simulink model "hw6_"  (Simulink 7.9)
settings: Solver=ode45  StartTime=0.0  StopTime=200.0  RelTol=1e-3
settings Model: Creator=bazkoale  LastModifiedBy=alex
settings DataIOCC: SignalLoggingSaveFormat=Dataset
settings OptimizationCC: ExpressionDepthLimit=128
settings DebuggingCC: MultiTaskDSMMsg=warning  MultiTaskCondExecSysMsg=none  StrictBusMsg=None
settings RTWCC: IncludeERTFirstTime=on
settings CodeAppCC: CustomSymbolStrType=$N$R$M_T

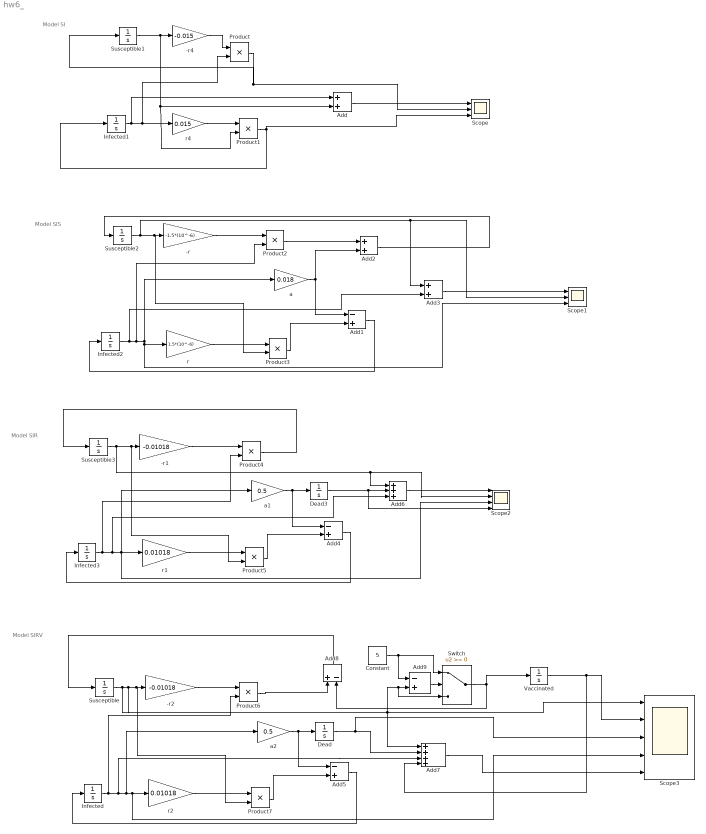
== system hw6_ ==
  note: Model SI
  note: Model SIS
  note: Model SIR
  note: Model SIRV
  -r : Gain  Gain=-1.5*(10^-6)
  -r1 : Gain  Gain=-0.01018
  -r2 : Gain  Gain=-0.01018
  -r4 : Gain  Gain=-0.015
  Add : Sum
  Add{1,4..5,9} (4 alike) : Sum  Inputs=-+
  Add2 : Sum
  Add3 : Sum
  Add6 : Sum  Inputs=+++
  Add7 : Sum  Inputs=++++
  Add8 : Sum  Inputs=+-
  Constant : Constant  Value=5
  Dead : Integrator
  Dead3 : Integrator
  Infected : Integrator  InitialCondition=1
  Infected1 : Integrator  InitialCondition=1
  Infected2 : Integrator  InitialCondition=10
  Infected3 : Integrator  InitialCondition=1
  Product{,1..7} (8 alike) : Product
  Scope : Scope  NumInputPorts=3
      settings: YMin=-5~-5~-5  YMax=5~5~5
  Scope1 : Scope  NumInputPorts=3
      settings: YMin=-5~-5~-5  YMax=5~5~5
  Scope2 : Scope  NumInputPorts=4
      settings: YMin=-5~-5~-5~-5  YMax=5~5~5~5  SaveName=ScopeData2
  Scope3 : Scope  NumInputPorts=5
      settings: YMin=-5~-5~-5~-5~-5  YMax=5~5~5~5~5  SaveName=ScopeData3
  Susceptible : Integrator  InitialCondition=99
  Susceptible1 : Integrator  InitialCondition=99
  Susceptible2 : Integrator  InitialCondition=200000-10
  Susceptible3 : Integrator  InitialCondition=99
  Switch : Switch
  Vaccinated : Integrator
  a : Gain  Gain=0.018
  a1 : Gain  Gain=0.5
  a2 : Gain  Gain=0.5
  r : Gain  Gain=1.5*(10^-6)
  r1 : Gain  Gain=0.01018
  r2 : Gain  Gain=0.01018
  r4 : Gain  Gain=0.015
  wires:
  Susceptible1/1 -> Add/2, Product1/2, -r4/1
  Infected1/1 -> Add/1, Product/2, r4/1
  Product/1 -> Scope/2, Susceptible1/1
  Product1/1 -> Infected1/1, Scope/3
  Add/1 -> Scope/1
  -r4/1 -> Product/1
  r4/1 -> Product1/1
  Susceptible2/1 -> Scope1/2, Add3/1, Product3/2, -r/1
  Infected2/1 -> Add3/2, Scope1/3, r/1, a/1, Product2/2
  -r/1 -> Product2/1
  r/1 -> Product3/1
  Product2/1 -> Add2/1
  a/1 -> Add1/1, Add2/2
  Add2/1 -> Susceptible2/1
  Product3/1 -> Add1/2
  Add1/1 -> Infected2/1
  Add3/1 -> Scope1/1
  Susceptible3/1 -> -r1/1, Product5/2, Add6/1, Scope2/2
  Infected3/1 -> Add6/3, Scope2/3, r1/1, a1/1, Product4/2
  -r1/1 -> Product4/1
  r1/1 -> Product5/1
  Product4/1 -> Susceptible3/1
  a1/1 -> Dead3/1, Add4/1
  Product5/1 -> Add4/2
  Add4/1 -> Infected3/1
  Add6/1 -> Scope2/1
  Dead3/1 -> Add6/2, Scope2/4
  Susceptible/1 -> Product7/2, -r2/1, Scope3/1, Add7/1, Add9/2, Switch/3
  -r2/1 -> Product6/1
  r2/1 -> Product7/1
  a2/1 -> Add5/1, Dead/1
  Product7/1 -> Add5/2
  Dead/1 -> Scope3/3, Add7/2
  Switch/1 -> Add8/2, Vaccinated/1
  Product6/1 -> Add8/1
  Add8/1 -> Susceptible/1
  Vaccinated/1 -> Add7/4, Scope3/2
  Add5/1 -> Infected/1
  Infected/1 -> Product6/2, a2/1, Scope3/4, r2/1, Add7/3
  Add7/1 -> Scope3/5
  Add9/1 -> Switch/2
  Constant/1 -> Switch/1, Add9/1
